simulink model "VB_Fahrzeug_Acc"  (Simulink 4.00)
settings: Solver=ode5  StartTime=0.0  StopTime=1  FixedStep=0.01  RelTol=1e-3
values from neighbouring files (symbols this model uses):
  drive_acc =     [NoGenDoubleNEDC.mat]
  IGen = KonstantLeerlaufStrom    [DPVorwaerts_TrajMatBC.m]    (also in TrajMatAufbau.m = KonstantLeerlaufStrom*ones(size([0:USchritt:Umax])))
  ILoad = 12    [TrajMatBauRun.m]
  LadungAnfang = InitialCharge    [DPVorwaerts_TrajMatBC.m]
  lm_alternator =     [NoGenDoubleNEDC.mat]
  nom_cap = 65    [AGM_ini_file.m]
  PwpPt_Tq_EngGross = [0 0 0 1.18647349782e-14 1.38134887733e-14 1.57622425684e-14 1.77109963635e-14 1.96597501586e-14 2.16085039538e-14 2.35572577489e-14 2.5506011544e-14 2.74547653391e-14 ... (23602 elements, 23602x1)]    [NoGenDoubleNEDC.mat]    (also in newdoublecycle.m = [PwpPt_Tq_EngGross;PwpPt_Tq_EngGross])
  PwpPt_W_EngDn = [750 750 750 750 750 750 750 750 750 750 750 750 ... (23602 elements, 23602x1)]    [NoGenDoubleNEDC.mat]    (also in newdoublecycle.m = [PwpPt_W_EngDn;PwpPt_W_EngDn])
  sim_sample_time = [0 0.1 0.2 0.3 0.4 0.5 0.6 0.7 0.8 0.9 1 1.1 ... (23602 elements, 23602x1)]    [NoGenDoubleNEDC.mat]    (also in newdoublecycle.m = [sim_sample_time;sim_sample_time+max(sim_sample_time)+0.1])
  SOC_beg = 70    [AGM_ini_file.m]    (also in DP_Batt_Init.m = battery.init_SOC)
  T0 = k-1+StartZeit    [DPRueck_TrajMatBC.m]    (also in DPVorwaerts_TrajMatBC.m; TrajMatAufbau.m = k-1)
  Xmax = 5.0    (= 5)    [DPTrajMatBCRun.m]
  Xmin = -5.0    (= -5)    [DPTrajMatBCRun.m]
settings Model: LastModifiedBy=meifert  SimulationMode=accelerator

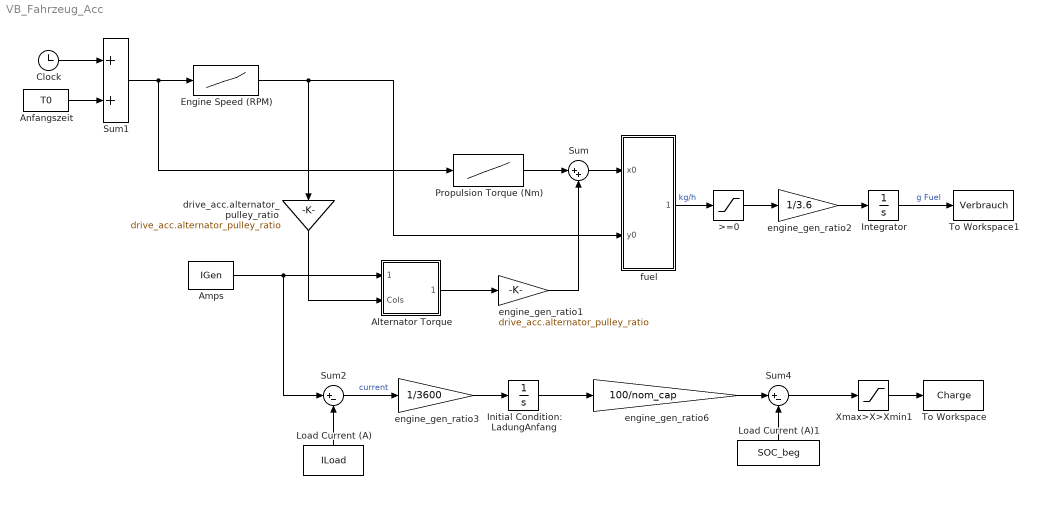
== system VB_Fahrzeug_Acc ==
  >=0 : Saturate  UpperLimit=inf  LowerLimit=0  LinearizeAsGain=on
  Alternator Torque : Subsystem  AncestorBlock=|  mask(Lookup Table (2-D)){x=lm_alternator.amp, y=lm_alternator.rpm, t=lm_alternator.loss}
      | simulink3/Functions
      | & Tables/Look-Up
      | Table (2-D)
      mask prompts: x "Row:"; y "Column:"; t "Table:"
      mask help: Performs 2-D linear interpolation of input values using the specified input/output table. Extrapolation is performed outside the table boundaries. The first dimension corresponds to the top (or left) input port.
      mask init:
      | [r,c]=size(t);
      | xt=reshape(x,prod(size(x)),1);
      | xi=xt(:,ones(1,c));
      | minx=min(x); maxx=max(x);
      | mint=min(min(t)); maxt=max(max(t));
      settings: RTWFcnNameOpts=Auto  RTWFileNameOpts=Auto
      mask Display: plot(double(xi),double(t),double([minx maxx]),double([mint mint]),double([minx minx]),double([mint maxt]))
  Amps : Constant  Value=IGen
  Anfangszeit : Constant  Value=T0
  Clock : Clock
      settings: DisplayTime=off  Decimation=10
  Engine Speed (RPM) : Lookup  InputValues=sim_sample_time  OutputValues=PwpPt_W_EngDn
  Initial Condition: LadungAnfang : Integrator  ExternalReset=none  InitialConditionSource=internal  InitialCondition=LadungAnfang*nom_cap/100  LimitOutput=off  UpperSaturationLimit=inf  LowerSaturationLimit=-inf  ShowSaturationPort=off  ShowStatePort=off  AbsoluteTolerance=auto
  Integrator : Integrator  ExternalReset=none  InitialConditionSource=internal  InitialCondition=0  LimitOutput=off  UpperSaturationLimit=inf  LowerSaturationLimit=-inf  ShowSaturationPort=off  ShowStatePort=off  AbsoluteTolerance=auto
  Load Current (A) : Constant  Orientation=up  Value=ILoad
  Load Current (A)1 : Constant  Orientation=up  Value=SOC_beg
  Propulsion Torque (Nm) : Lookup  InputValues=sim_sample_time  OutputValues=PwpPt_Tq_EngGross
  Sum : Sum  Inputs=|++  SaturateOnIntegerOverflow=on
  Sum1 : Sum  Inputs=++  SaturateOnIntegerOverflow=on
  Sum2 : Sum  Inputs=|+-  SaturateOnIntegerOverflow=on
  Sum4 : Sum  Inputs=|+-  SaturateOnIntegerOverflow=on
  To Workspace : ToWorkspace  VariableName=Charge  SampleTime=-1  SaveFormat=Array
  To Workspace1 : ToWorkspace  VariableName=Verbrauch  SampleTime=-1  SaveFormat=Array
  Xmax>X>Xmin1 : Saturate  UpperLimit=Xmax  LowerLimit=Xmin  LinearizeAsGain=on
  drive_acc.alternator_pulley_ratio : Gain  Orientation=down  Gain=drive_acc.alternator_pulley_ratio  Multiplication=Element-wise(K.*u)  SaturateOnIntegerOverflow=on
  engine_gen_ratio1 : Gain  Gain=drive_acc.alternator_pulley_ratio  Multiplication=Element-wise(K.*u)  SaturateOnIntegerOverflow=on
  engine_gen_ratio2 : Gain  Gain=1/3.6  Multiplication=Element-wise(K.*u)  SaturateOnIntegerOverflow=on
  engine_gen_ratio3 : Gain  Gain=1/3600  Multiplication=Element-wise(K.*u)  SaturateOnIntegerOverflow=on
  engine_gen_ratio6 : Gain  Gain=100/nom_cap  Multiplication=Element-wise(K.*u)  SaturateOnIntegerOverflow=on
  fuel : Subsystem  mask(2-D Table Lookup){@1=engine.tq, @2=engine.rpm, @3=engine.fuel}
      mask prompts: @1 "X Index"; @2 "Y Index"; @3 "Table"
      mask help:
      | Two Dimensional Table Lookup
      | The first input corresponds to X Index and the second input corresponds to the Y Index
      mask init:
      | xindex=@1; yindex=@2; table=@3; sftab2chk(xindex,yindex,table);
      settings: RTWFcnNameOpts=Auto  RTWFileNameOpts=Auto
      mask Help: This block returns a linearly interpolated intersection from the table using the X index (which corresponds to the rows of the table) and the Y index (which corresponds to the columns of the table).  Extrapolation is used.
      mask Display: plot(-10,-10,110,110,[90,50,10],[90,40,30],[90,50,10],[50,26,20],[90,50,10],[22,13,10])
  wires:
  Integrator/1 -> To Workspace1/1  "g Fuel"
  fuel/1(table out) -> >=0/1  "kg/h"
  >=0/1 -> engine_gen_ratio2/1
  Anfangszeit/1 -> Sum1/2
  Clock/1 -> Sum1/1
  Sum1/1 -> Engine Speed (RPM)/1, Propulsion Torque (Nm)/1
  Engine Speed (RPM)/1 -> drive_acc.alternator_pulley_ratio/1, fuel/2(y0)
  Alternator Torque/1(Out1) -> engine_gen_ratio1/1
  Amps/1 -> Sum2/1, Alternator Torque/1(Rows)
  engine_gen_ratio1/1 -> Sum/2
  Load Current (A)/1 -> Sum2/2
  Propulsion Torque (Nm)/1 -> Sum/1
  engine_gen_ratio2/1 -> Integrator/1
  drive_acc.alternator_pulley_ratio/1 -> Alternator Torque/2(Cols)
  Sum/1 -> fuel/1(x0)
  Sum2/1 -> engine_gen_ratio3/1  "current"
  engine_gen_ratio3/1 -> Initial Condition: LadungAnfang/1
  Xmax>X>Xmin1/1 -> To Workspace/1
  Load Current (A)1/1 -> Sum4/2
  Sum4/1 -> Xmax>X>Xmin1/1
  Initial Condition: LadungAnfang/1 -> engine_gen_ratio6/1
  engine_gen_ratio6/1 -> Sum4/1

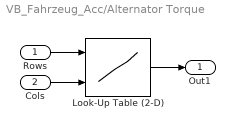
== system VB_Fahrzeug_Acc/Alternator Torque ==
  Rows : Inport  Port=1
  Cols : Inport  Port=2
  Look-Up Table (2-D) : Lookup2D  RowIndex=x  ColumnIndex=y  OutputValues=t
  Out1 : Outport  Port=1
  wires:
  Rows/1 -> Look-Up Table (2-D)/1
  Cols/1 -> Look-Up Table (2-D)/2
  Look-Up Table (2-D)/1 -> Out1/1

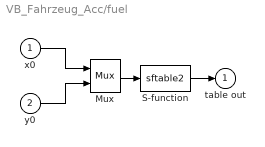
== system VB_Fahrzeug_Acc/fuel ==
  x0 : Inport  Port=1
  y0 : Inport  Port=2
  Mux : Mux  Inputs=2
      settings: DisplayOption=none
  S-function : S-Function  FunctionName=sftable2  Parameters=xindex, yindex, table  PortCounts=[]  SFunctionModules=''
  table out : Outport  Port=1  InitialOutput=0
  wires:
  Mux/1 -> S-function/1
  x0/1 -> Mux/1
  S-function/1 -> table out/1
  y0/1 -> Mux/2
